simulink model "Copy_2_of_motor_new"  (R2018b)
settings: Solver=FixedStepAuto  StartTime=0.0  StopTime=100  FixedStep=0.001  RelTol=1e-3
values from neighbouring files (symbols this model uses):
  wc = 20    [Para_new.m]
  wt = 20    [Para_new.m]
settings Model: Creator=chengqian  LastModifiedBy=chengqian
settings SolverCC: AlgebraicLoopSolver=LineSearch

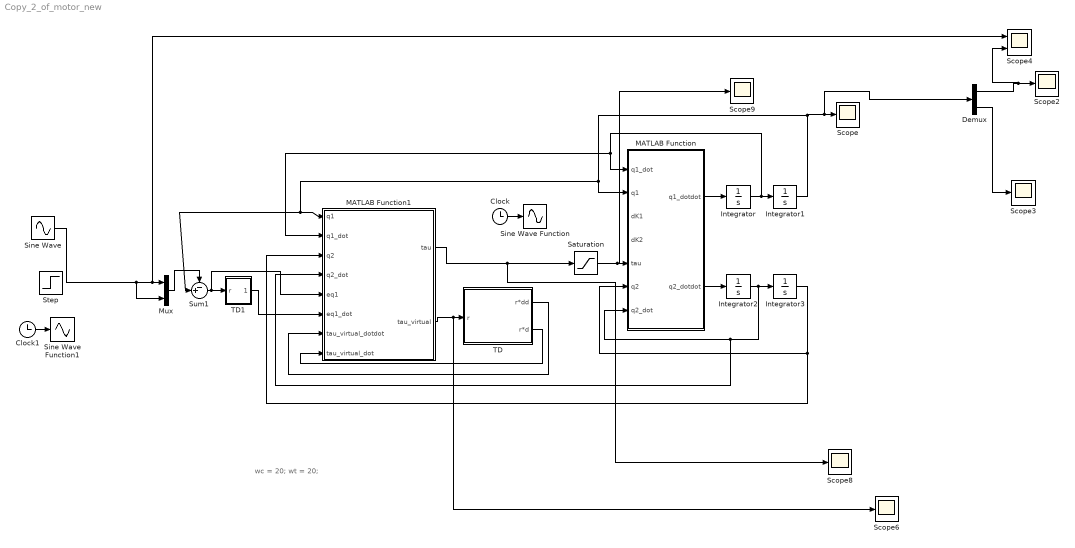
== system Copy_2_of_motor_new ==
  note: wc = 20;
      | wt = 20;
  Clock : Clock
  Clock1 : Clock
  Demux : Demux  Outputs=2
  Integrator{,1..3} (4 alike) : Integrator
  MATLAB Function : MATLAB Function  TreatAsAtomicUnit=on
  MATLAB Function1 : MATLAB Function  TreatAsAtomicUnit=on
  Mux : Mux  Inputs=2
  Saturation : Saturate  UpperLimit=[1000;1000]  LowerLimit=-[1000;1000]
  Scope{,2..3,6,8..9} (6 alike) : Scope
  Scope4 : Scope  NumInputPorts=2
  Sine Wave : Sin  Amplitude=0.1  Frequency=0.5  SampleTime=0
  Sine Wave Function : Sin  TimeSource=Use external signal  Amplitude=0.4  Frequency=20  SampleTime=0
  Sine Wave Function1 : Sin  TimeSource=Use external signal  Amplitude=0.4  Frequency=20  SampleTime=0
  Step : Step  Time=0  After=0.1  SampleTime=0
  Sum1 : Sum  Inputs=-+|
  TD : Subsystem
  TD1 : Subsystem
  wires:
  MATLAB Function1/2(tau_virtual) -> Scope6/1, TD/1(r)
  MATLAB Function/1(q1_dotdot) -> Integrator/1
  Integrator/1 -> MATLAB Function/1(q1_dot), MATLAB Function1/2(q1_dot), Integrator1/1
  Integrator2/1 -> MATLAB Function1/4(q2_dot), MATLAB Function/7(q2_dot), Integrator3/1
  MATLAB Function/2(q2_dotdot) -> Integrator2/1
  Integrator3/1 -> MATLAB Function/6(q2), MATLAB Function1/3(q2)
  Clock/1 -> Sine Wave Function/1
  TD/2(r*d) -> MATLAB Function1/8(tau_virtual_dot)
  TD/1(r*dd) -> MATLAB Function1/7(tau_virtual_dotdot)
  Sum1/1 -> TD1/1(r), MATLAB Function1/5(eq1)
  Mux/1 -> Sum1/1
  MATLAB Function1/1(tau) -> Saturation/1, Scope8/1
  Saturation/1 -> Scope9/1, MATLAB Function/5(tau)
  Demux/2 -> Scope3/1
  TD1/1(r*d) -> MATLAB Function1/6(eq1_dot)
  Clock1/1 -> Sine Wave Function1/1
  Sine Wave/1 -> Mux/2, Scope4/1, Mux/1
  Integrator1/1 -> Demux/1, Scope/1, Sum1/2, MATLAB Function1/1(q1), MATLAB Function/2(q1)
  Demux/1 -> Scope4/2, Scope2/1

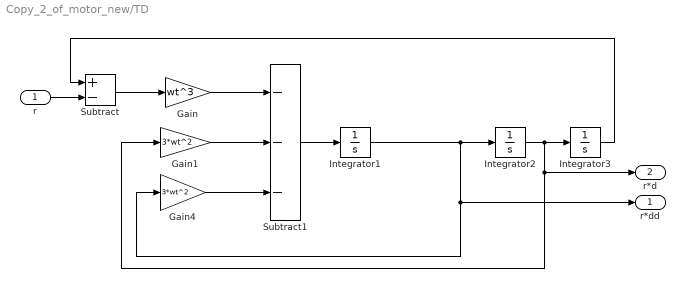
== system Copy_2_of_motor_new/TD ==
  r : Inport
  Gain : Gain  Gain=wt^3
  Gain1 : Gain  Gain=3*wt^2
  Gain4 : Gain  Gain=3*wt^2
  Integrator1 : Integrator
  Integrator2 : Integrator
  Integrator3 : Integrator
  Subtract : Sum  Inputs=+-
  Subtract1 : Sum  Inputs=---
  r*dd : Outport
  r*d : Outport  Port=2
  wires:
  Integrator2/1 -> Integrator3/1, Gain1/1, r*d/1
  Gain1/1 -> Subtract1/2
  Subtract/1 -> Gain/1
  Gain/1 -> Subtract1/1
  Integrator3/1 -> Subtract/1
  Gain4/1 -> Subtract1/3
  Subtract1/1 -> Integrator1/1
  Integrator1/1 -> Gain4/1, r*dd/1, Integrator2/1
  r/1 -> Subtract/2

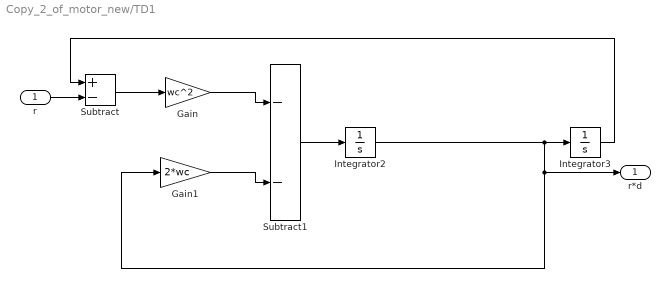
== system Copy_2_of_motor_new/TD1 ==
  r : Inport
  Gain : Gain  Gain=wc^2
  Gain1 : Gain  Gain=2*wc
  Integrator2 : Integrator
  Integrator3 : Integrator
  Subtract : Sum  Inputs=+-
  Subtract1 : Sum  Inputs=--
  r*d : Outport
  wires:
  Integrator2/1 -> Integrator3/1, Gain1/1, r*d/1
  Gain1/1 -> Subtract1/2
  Subtract/1 -> Gain/1
  Gain/1 -> Subtract1/1
  Subtract1/1 -> Integrator2/1
  r/1 -> Subtract/2
  Integrator3/1 -> Subtract/1

== matlab function Copy_2_of_motor_new/MATLAB Function1 ==
  data: q1 input; tau output size=2; q1_dot input; q2 input; q2_dot input; eq1 input; eq1_dot input; tau_virtual_dotdot input; tau_virtual_dot input; tau_virtual output size=2
function [tau,tau_virtual] = fcn(q1,q1_dot,q2,q2_dot,eq1,eq1_dot,tau_virtual_dotdot,tau_virtual_dot)

J11 = 3.17*10^(-4);
J22 = 0.97*10^(-4);
I1 = 0.96;
I2 = 0.71;
l1 = 0.6;
lc1 = 0.3;
lc2 = 0.5;
m1 = 19.31;
m2 = 13.73;
K1_ = 1.06*10^3;
K2_ = 0.75*10^3;
g = 9.8;

S11 = 1;
S12 = 1;
S21 = 2;
S22 = 2;
w1 =1;
beta1 = 2; beta2 = 2;
alpha1 = 10; alpha2 = 10;
Kp1 = 100; Kd1 =20;

dK1=0;dK2=0;

q11 = q1(1);
q12 = q1(2);
q11_dot = q1_dot(1);
q12_dot = q1_dot(2);

q21 = q2(1);
q22 =q2(2);
q21_dot = q2_dot(1);
q22_dot = q2_dot(2);

M11 = m2*(l1^2 + lc2^2 + 2*l1*lc2*cos(q12)) + m1*lc1^2 + I1 + I2;
M12 = m2*(lc2^2 + l1*lc2*cos(q12)) + I2;
M21 = M12;
M22 = m2*lc2^2 + I2;

M = [M11,M12;M21,M22];

C11 = -m1*l1*lc2*sin(q12)*q12_dot;
C12 = -m2*l1*lc2*sin(q12)*(q11_dot + q12_dot);
C21 = m2*l1*lc2*sin(q12)*q11_dot;
C22 = 0;

Kp2 = 400;
Kd2 = 200;

C = [C11,C12;C21,C22];

G1 = (m1*lc1 + m2*l1)*g*sin(q11) + m2*lc2*g*sin(q11 + q12);
G2 = m2*lc2*g*sin(q11+q12);

G = [G1;G2];

J = diag([J11,J22]);
S1 = diag([S11,S12]);
S2 = diag([S21,S22]);
K_ = diag([K1_,K2_]);
K = diag([K1_,K2_])*(eye(2) + diag([dK1,dK2]));

M11_dot = -2*m2*l1*lc2*sin(q12)*q12_dot;
M12_dot = -m2*l1*lc2*sin(q12)*q12_dot;
M21_dot = -m2*l1*lc2*sin(q11)*q12_dot;
M22_dot = 0;

M_dot = [M11_dot,M12_dot;M21_dot,M22_dot];

PHI1 = 0.5*M_dot*(q1_dot + S1*q1) - C*q1_dot - G -K_*q1 + M*S1*q1_dot;
rol1_bound = norm(PHI1);
rol1 = rol1_bound;


tau_virtual =(K_'*(-alpha1*(eq1_dot + S1*eq1)*rol1^2 - beta1*(eq1_dot + S1*eq1)) + K_'*(-Kp1*eq1 - Kd1*eq1_dot));
%tau_virtual =K_'* u1;% (K_'*(-alpha1*(q1_dot + S1*q1)*rol1^2 - beta1*(q1_dot + S1*q1)) + K_'*(Kp1*q1_r - Kp1*q1 - Kd1*q1_dot));+ 
x3 = q2 - tau_virtual;
x4 = q2_dot - tau_virtual_dot;
PHI2 = -J*tau_virtual_dotdot - K_*(x3) + K_*q1 - K_*tau_virtual + J*S2*x4;
rol2_bound = norm(PHI2);
rol2 = rol2_bound;


tau =(-alpha2*(x4+S2*x3)*rol2^2 - beta2*(x4+S2*x3));
%q2_dotdot_dd = J'*(tau + K*(q1_d - q2_d));

== matlab function Copy_2_of_motor_new/MATLAB Function ==
  data: q1_dot input; q1 input; dK1 input; dK2 input; q1_dotdot output size=2; tau input; q2 input; q2_dot input; q2_dotdot output size=2
function [q1_dotdot,q2_dotdot] = fcn(q1_dot,q1,dK1,dK2,tau,q2,q2_dot)
J11 = 3.17*10^(-4);
J22 = 0.97*10^(-4);
I1 = 0.96;
I2 = 0.71;
l1 = 0.6;
lc1 = 0.3;
lc2 = 0.5;
m1 = 19.31;
m2 = 13.73;
K1_ = 1.06*10^3;
K2_ = 0.75*10^3;
g = 9.8;

S11 = 1;
S12 = 1;
S21 = 2;
S22 = 2;
w1 =1;
beta1 = 2; beta2 = 2;
alpha1 = 10; alpha2 = 10;
Kp1 = 100; Kd1 =20;


q11 = q1(1);
q12 = q1(2);
q11_dot = q1_dot(1);
q12_dot = q1_dot(2);

q21 = q2(1);
q22 =q2(2);
q21_dot = q2_dot(1);
q22_dot = q2_dot(2);

M11 = m2*(l1^2 + lc2^2 + 2*l1*lc2*cos(q12)) + m1*lc1^2 + I1 + I2;
M12 = m2*(lc2^2 + l1*lc2*cos(q12)) + I2;
M21 = M12;
M22 = m2*lc2^2 + I2;

M = [M11,M12;M21,M22];

C11 = -m1*l1*lc2*sin(q12)*q12_dot;
C12 = -m2*l1*lc2*sin(q12)*(q11_dot + q12_dot);
C21 = m2*l1*lc2*sin(q12)*q11_dot;
C22 = 0;

C = [C11,C12;C21,C22];

G1 = (m1*lc1 + m2*l1)*g*sin(q11) + m2*lc2*g*sin(q11 + q12);
G2 = m2*lc2*g*sin(q11+q12);

G = [G1;G2];

J = diag([J11,J22]);
S1 = diag([S11,S12]);
S2 = diag([S21,S22]);
K = diag([K1_,K2_])*(eye(2) + diag([dK1,dK2]));

q1_dotdot = -M'*(C*q1_dot + G + K*(q1-q2));
q2_dotdot = J'*(tau + K*(q1-q2));
